simulink model "mcb_pmsm_foc_qep_dyno_f28069m_ADC"  (R2023b)
settings: Solver=FixedStepDiscrete  StartTime=0.0  StopTime=4  RelTol=1e-3  EnableMultiTasking=on
InitFcn:
  | mcb_pmsm_foc_qep_dyno_f28069m_data;
undefined symbols (not defined in the file): DiscIntNeverNeededParam, Down, GPTRIP1SEL, GPTRIP2SEL, inverter_motor1, inverter_motor2, PI_params_motor1, PI_params_motor2, pmsm_motor1, pmsm_motor2, PU_System_motor2, target, Ts, Ts_motor, Ts_speed, TZ1, TZ2, Up
libraries: c2802xlib x12, simulink x11, c280xlib x8, mcbcontrolslib x6, mcbpositiondecoderlib x6, c2806xlib x5, svdschedulerlib x3, mcbpmsmnonlinearlib x2, autolibpmsmexterior x2, mcbplantlib x2, demo_controls x1, slpidlib x1
(part 3 of 4)

== system mcb_pmsm_foc_qep_dyno_f28069m_ADC/Serial Receive/Code Generation ==
  SCI Receive : c280xlib/SCI Receive  sciModule=A  dataHead=''  headerCheckMaxCount=16  dataTail=''  dataType=uint16  dataLenOptions=Length via dialog  dataDim=2  maxDataLength=1  initValue=0  errOption=Output the last received value  errValue=0  sampleTime=-1  blockingMode=on  timeOut=0.019444  outputStatus=off
  Data : Outport
  wires:
  SCI Receive/1 -> Data/1

== system mcb_pmsm_foc_qep_dyno_f28069m_ADC/Serial Receive/Reference Signal ==
  In1 : Inport
  Data Store Write2 : DataStoreWrite  DataStoreName=Debug_signals  IndexOptions=Index vector (dialog)  Indices=1  OutputSizes=1
  Data_Conditioning : Subsystem
  If : If  IfExpression=u1 == 1  ElseIfExpressions=u1 == 2, u1 == 0  ShowElse=off
  If Action Subsystem : Subsystem  TreatAsAtomicUnit=on
  If Action Subsystem1 : Subsystem  TreatAsAtomicUnit=on
  If Action Subsystem2 : Subsystem  TreatAsAtomicUnit=on
  unParse : Subsystem
  Enable_PWM : Outport
  wires:
  If/3 -> If Action Subsystem2/Action
  unParse/3(Debug_sig) -> Data Store Write2/1
  Data_Conditioning/2(PU_data) -> If Action Subsystem2/1(In1), If Action Subsystem/1(In1), If Action Subsystem1/1(In1)
  If/2 -> If Action Subsystem1/Action
  If/1 -> If Action Subsystem/Action
  In1/1 -> Data_Conditioning/1(In1)
  unParse/2(Motor1/2) -> If/1
  Data_Conditioning/1(Logical signal) -> unParse/1(Data)
  unParse/1(Enable_PWM) -> Enable_PWM/1

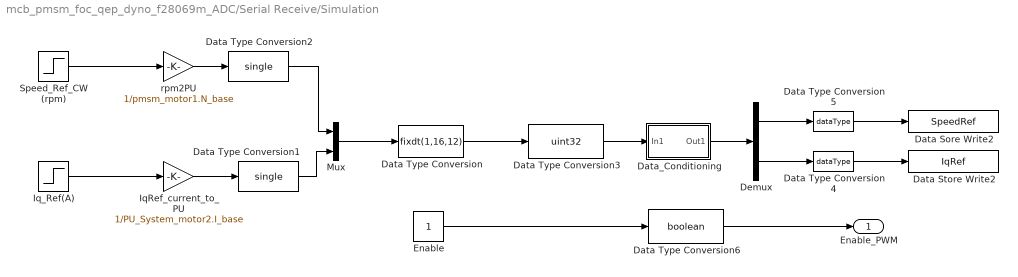
== system mcb_pmsm_foc_qep_dyno_f28069m_ADC/Serial Receive/Simulation ==
  Data Sore Write2 : DataStoreWrite  DataStoreName=SpeedRef  IndexOptions=Index vector (dialog)  Indices=1  OutputSizes=1
  Data Store Write2 : DataStoreWrite  DataStoreName=IqRef  IndexOptions=Index vector (dialog)  Indices=1  OutputSizes=1
  Data Type Conversion : DataTypeConversion  OutDataTypeStr=fixdt(1,16,12)  RndMeth=Simplest  SaturateOnIntegerOverflow=off
  Data Type Conversion1 : DataTypeConversion  OutDataTypeStr=single  RndMeth=Simplest  SaturateOnIntegerOverflow=off
  Data Type Conversion2 : DataTypeConversion  OutDataTypeStr=single  RndMeth=Simplest  SaturateOnIntegerOverflow=off
  Data Type Conversion3 : DataTypeConversion  OutDataTypeStr=uint32  ConvertRealWorld=Stored Integer (SI)  RndMeth=Simplest  SaturateOnIntegerOverflow=off
  Data Type Conversion4 : DataTypeConversion  OutDataTypeStr=dataType  RndMeth=Simplest  SaturateOnIntegerOverflow=off
  Data Type Conversion5 : DataTypeConversion  OutDataTypeStr=dataType  RndMeth=Simplest  SaturateOnIntegerOverflow=off
  Data Type Conversion6 : DataTypeConversion  OutDataTypeStr=boolean  SaturateOnIntegerOverflow=off  RndMeth=Floor
  Data_Conditioning : Subsystem
  Demux : Demux  Outputs=2
  Enable : Constant  OutDataTypeStr=single
  IqRef_current_to_PU : Gain  Gain=1/PU_System_motor2.I_base  RndMeth=Simplest  OutDataTypeStr=Inherit: Same as input
  Iq_Ref(A) : Step  Time=3  Before=1  After=0.8*pmsm_motor2.I_rated  OutDataTypeStr=single
  Mux : Mux  Inputs=2
  Speed_Ref_CW (rpm) : Step  Before=0.2*pmsm_motor1.N_base  After=0.5*pmsm_motor1.N_base  OutDataTypeStr=single
  rpm2PU : Gain  Gain=1/pmsm_motor1.N_base  RndMeth=Simplest  OutDataTypeStr=Inherit: Same as input
  Enable_PWM : Outport
  wires:
  Data Type Conversion3/1 -> Data_Conditioning/1(In1)
  rpm2PU/1 -> Data Type Conversion2/1
  Data Type Conversion1/1 -> Mux/2
  Data Type Conversion2/1 -> Mux/1
  Data Type Conversion/1 -> Data Type Conversion3/1
  Mux/1 -> Data Type Conversion/1
  Speed_Ref_CW (rpm)/1 -> rpm2PU/1
  IqRef_current_to_PU/1 -> Data Type Conversion1/1
  Iq_Ref(A)/1 -> IqRef_current_to_PU/1
  Data_Conditioning/1(Out1) -> Demux/1
  Demux/1 -> Data Type Conversion5/1
  Data Type Conversion4/1 -> Data Store Write2/1
  Demux/2 -> Data Type Conversion4/1
  Data Type Conversion5/1 -> Data Sore Write2/1
  Data Type Conversion6/1 -> Enable_PWM/1
  Enable/1 -> Data Type Conversion6/1

== system mcb_pmsm_foc_qep_dyno_f28069m_ADC/Simulation/Simulation1 ==
  Trigger : TriggerPort  VariantControl=Variant  PortDimensions=1
  ADCINT1 : simulink/Ports & Subsystems/Function-Call Generator  sample_time=-1  numberOfIterations=1  DisallowWideOutput=off
  Interrupt : Outport
  wires:
  ADCINT1/1 -> Interrupt/1

== system mcb_pmsm_foc_qep_dyno_f28069m_ADC/Simulation/Simulation2 ==
  Trigger : TriggerPort  VariantControl=Variant  PortDimensions=1
  ADCINT1 : simulink/Ports & Subsystems/Function-Call Generator  sample_time=-1  numberOfIterations=1  DisallowWideOutput=off
  Interrupt : Outport
  wires:
  ADCINT1/1 -> Interrupt/1

== system mcb_pmsm_foc_qep_dyno_f28069m_ADC/Speed Control for motor1/PI_Controller_Speed ==
  N_ref : Inport
  N_fb : Inport  Port=2
  AND : Logic  IconShape=distinctive  AllPortsSameDT=off  OutDataTypeStr=boolean
  Data Store Read1 : DataStoreRead  DataStoreName=Enable  IndexOptions=Index vector (dialog)  Indices=1  OutputSizes=1
  Data Store Read2 : DataStoreRead  DataStoreName=EnClosedLoop  IndexOptions=Index vector (dialog)  Indices=1  OutputSizes=1
  Discrete PI Controller with anti-windup & reset : slpidlib/PID Controller  Controller=PI  Form=Parallel  TimeDomain=Discrete-time  UseExternalTs=off  SampleTime=-1  IntegratorMethod=Forward Euler  FilterMethod=Forward Euler  ControllerParametersSource=external  P=1  I=1  UseKiTs=on  D=0  N=100  UseFilter=on  TunerSelectOption=Transfer Function Based (PID Tuner App)  InitialConditionSource=external  InitialConditionForIntegrator=0  InitialConditionForFilter=0  DifferentiatorICPrevScaledInput=0  ExternalReset=level  TrackingMode=off  Kt=1  LimitOutput=on  SatLimitsSource=internal  UpperSaturationLimit=1  LowerSaturationLimit=-1  LinearizeAsGain=on  AntiWindupMode=clamping  Kb=1  LimitIntegrator=off  UpperIntegratorSaturationLimit=inf  LowerIntegratorSaturationLimit=-inf  RndMeth=Simplest  POutMin=[]  POutMax=[]  IOutMin=[]  IOutMax=[]  DOutMin=[]  DOutMax=[]  NOutMin=[]  NOutMax=[]  SumOutMin=[]  SumOutMax=[]  SaturationOutDataTypeStr=Inherit: Inherit via back propagation  SaturationOutMin=[]  SaturationOutMax=[]  PParamMin=[]  PParamMax=[]  IParamMin=[]  IParamMax=[]  DParamMin=[]  DParamMax=[]  NParamMin=[]  NParamMax=[]  KbParamMin=[]  KbParamMax=[]  KtParamMin=[]  KtParamMax=[]  KbOutMin=[]  KbOutMax=[]  KtOutMin=[]  KtOutMax=[]  IntegratorOutMin=[]  IntegratorOutMax=[]  FilterOutMin=[]  FilterOutMax=[]  SumI1OutMin=[]  SumI1OutMax=[]  SumI2OutMin=[]  SumI2OutMax=[]  SumI3OutMin=[]  SumI3OutMax=[]  SumI4OutMin=[]  SumI4OutMax=[]  SumDOutMin=[]  SumDOutMax=[]  DifferentiatorOutMin=[]  DifferentiatorOutMax=[]  FilterDiffOutCoefMin=[]  FilterDiffOutCoefMax=[]  ReciprocalOutMin=[]  ReciprocalOutMax=[]  SumDenOutMin=[]  SumDenOutMax=[]  SumNumOutMin=[]  SumNumOutMax=[]  DivideOutMin=[]  DivideOutMax=[]  UdiffTsProdOutMin=[]  UdiffTsProdOutMax=[]  NTsProdOutMin=[]  NTsProdOutMax=[]  UintegralTsProdOutMin=[]  UintegralTsProdOutMax=[]  UngainTsProdOutMin=[]  UngainTsProdOutMax=[]  ClampingZeroOutDataTypeStr=Inherit: Inherit via back propagation  ClampingZeroOutMin=[]  ClampingZeroOutMax=[]  FilterDenConstantOutDataTypeStr=Inherit: Inherit via back propagation  FilterDenConstantOutMin=[]  FilterDenConstantOutMax=[]  PCopyOutDataTypeStr=Inherit: Inherit via back propagation  PCopyOutMin=[]  PCopyOutMax=[]  NCopyOutDataTypeStr=Inherit: Inherit via back propagation  NCopyOutMin=[]  NCopyOutMax=[]  IntegratorContinuousStateAttributes=''  IntegratorStateMustResolveToSignalObject=off  IntegratorRTWStateStorageClass=Auto  FilterContinuousStateAttributes=''  FilterStateMustResolveToSignalObject=off  FilterRTWStateStorageClass=Auto  ParallelPVariant=ExternalParameters  IdealPVariant=Disabled  IVariant=ExternalParameters  DVariant=Disabled  IntegratorVariant=Discrete  SatVariant=Enabled  AWVariant=DiscClampingParallel  PCopyVariant=Disabled  TRVariant=Disabled  FdbkBlocksVariant=Forward  IdealPFdbkVariant=Disabled  SatFdbkVariant=Disabled  DerivativeFilterVariant=Disabled  NVariant=Disabled  NCopyVariant=Disabled_SignalSpec  FilterICVariant=Disabled  IntegratorICVariant=ExternalICs  ExternalResetVariant=ExternalReset  TRSumVariant=Passthrough  SumFdbkVariant=Disabled  SumVariant=Sum_PI  TsampFilterVariant=InternalTs  TsampNgainVariant=Passthrough  TsampIntegralVariant=Disabled_SignalSpec  ExternalSaturationOutDataTypeStr=Inherit: Same as second input
  Ki1 : Constant  Value=PI_params_motor1.Ki_speed*Ts_speed  OutDataTypeStr=dataType  SampleTime=-1
  Ki2 : Constant  Value=0  OutDataTypeStr=dataType  SampleTime=-1
  Kp1 : Constant  Value=PI_params_motor1.Kp_speed  OutDataTypeStr=dataType  SampleTime=-1
  Logical Operator : Logic  Operator=NOT  IconShape=distinctive  AllPortsSameDT=off  OutDataTypeStr=boolean
  Sum : Sum  Inputs=|+-  OutDataTypeStr=Inherit: Same as first input
  Iq_ref : Outport  VectorParamsAs1DForOutWhenUnconnected=off
  wires:
  Discrete PI Controller with anti-windup & reset/1 -> Iq_ref/1
  Ki1/1 -> Discrete PI Controller with anti-windup & reset/3
  Kp1/1 -> Discrete PI Controller with anti-windup & reset/2
  N_fb/1 -> Sum/2
  N_ref/1 -> Sum/1
  Sum/1 -> Discrete PI Controller with anti-windup & reset/1
  Logical Operator/1 -> Discrete PI Controller with anti-windup & reset/4
  Ki2/1 -> Discrete PI Controller with anti-windup & reset/5
  AND/1 -> Logical Operator/1
  Data Store Read1/1 -> AND/1
  Data Store Read2/1 -> AND/2

== system mcb_pmsm_foc_qep_dyno_f28069m_ADC/Speed Control for motor1/Speed_Ref_Selector ==
  Speed_Ref_In : Inport
  Speed_Ref_Open : Inport  Port=2
  Data Store Read : DataStoreRead  DataStoreName=EnClosedLoop  IndexOptions=Index vector (dialog)  Indices=1  OutputSizes=1
  IIR Filter : mcbcontrolslib/IIR Filter  VariantControl=Low Pass Filter  VariantSelect=Low-pass  Filter_constant=0.01  advancedSettings=off  Ts=50e-6  cutOff_freq=32.1525
  Switch : Switch  Criteria=u2 > Threshold  Threshold=0.5  SaturateOnIntegerOverflow=off  InputSameDT=off
  Speed_Ref_PU : Outport
  wires:
  IIR Filter/1 -> Speed_Ref_PU/1
  Switch/1 -> IIR Filter/1
  Data Store Read/1 -> Switch/2
  Speed_Ref_Open/1 -> Switch/3
  Speed_Ref_In/1 -> Switch/1

== system mcb_pmsm_foc_qep_dyno_f28069m_ADC/FOC Algorithm Motor1/Control_System/Closed loop Control ==
  Iab_meas_PU : Inport
  Pos_PU : Inport  Port=2
  Idq_ref_PU : Inport  Port=3
  EnablePWM : Inport  Port=4
  Enable : EnablePort
  Current Control : Subsystem  ReferencedSubsystem=current_control  Kpd=PI_params_motor1.Kp_i  Kid=PI_params_motor1.Ki_i*Ts  Kpq=PI_params_motor1.Kp_i  Kiq=PI_params_motor1.Ki_i*Ts
  Terminator : Terminator
  Vabc in PU : Outport
  Idq_debug : Outport  Port=2
  wires:
  Current Control/1 -> Vabc in PU/1
  Idq_ref_PU/1 -> Current Control/3
  EnablePWM/1 -> Current Control/4
  Current Control/2 -> Idq_debug/1
  Pos_PU/1 -> Current Control/2
  Iab_meas_PU/1 -> Current Control/1
  Current Control/3 -> Terminator/1

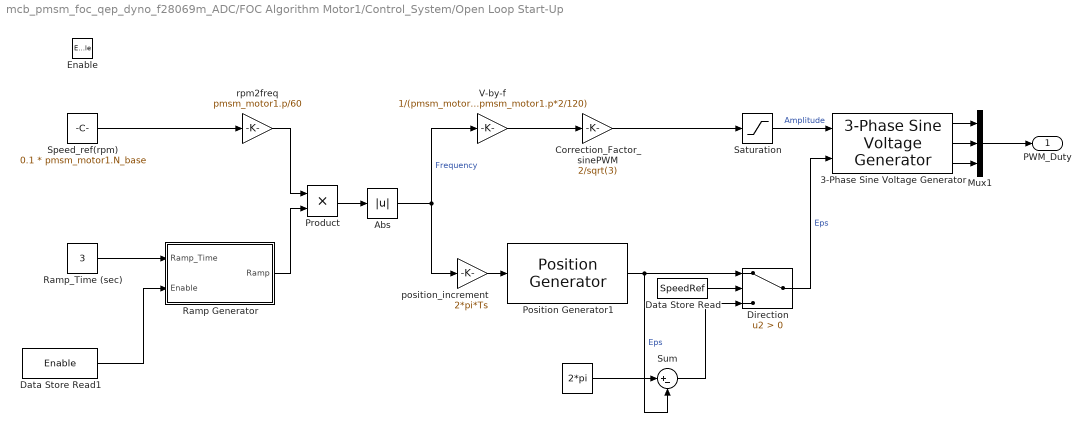
== system mcb_pmsm_foc_qep_dyno_f28069m_ADC/FOC Algorithm Motor1/Control_System/Open Loop Start-Up ==
  Enable : EnablePort
  " " : Constant  Value=2*pi  OutDataTypeStr=dataType  SampleTime=-1
  3-Phase Sine Voltage Generator : mcbcontrolslib/3-Phase Sine Voltage Generator  AngleInput=Radians  N_points=1024
  Abs : Abs  SaturateOnIntegerOverflow=off
  Correction_Factor_sinePWM : Gain  Gain=2/sqrt(3)  RndMeth=Simplest  OutDataTypeStr=Inherit: Same as input
  Data Store Read : DataStoreRead  DataStoreName=SpeedRef  IndexOptions=Index vector (dialog)  Indices=1  OutputSizes=1
  Data Store Read1 : DataStoreRead  DataStoreName=Enable  IndexOptions=Index vector (dialog)  Indices=1  OutputSizes=1
  Direction : Switch  Criteria=u2 > Threshold  OutDataTypeStr=dataType  RndMeth=Simplest  SaturateOnIntegerOverflow=off  InputSameDT=off
  Mux1 : Mux  Inputs=3
  Position Generator1 : mcbcontrolslib/Position Generator  AngleOutput=Radians  ExternalReset=none  Offset=0
  Product : Product  RndMeth=Simplest  OutDataTypeStr=Inherit: Same as first input
  Ramp Generator : Subsystem
  Ramp_Time (sec) : Constant  Value=3  OutDataTypeStr=dataType  SampleTime=-1
  Saturation : Saturate  UpperLimit=0.95  LowerLimit=0.15  RndMeth=Simplest
  Speed_ref(rpm) : Constant  Value=0.1 * pmsm_motor1.N_base  OutDataTypeStr=dataType  SampleTime=-1
  Sum : Sum  Inputs=|+-  RndMeth=Simplest  OutDataTypeStr=Inherit: Same as first input
  V-by-f : Gain  Gain=1/(pmsm_motor1.N_base*pmsm_motor1.p*2/120)  RndMeth=Simplest  OutDataTypeStr=Inherit: Same as input
  position_increment : Gain  Gain=2*pi*Ts  RndMeth=Simplest  OutDataTypeStr=Inherit: Same as input
  rpm2freq : Gain  Gain=pmsm_motor1.p/60  RndMeth=Simplest  OutDataTypeStr=Inherit: Same as input
  PWM_Duty : Outport  VectorParamsAs1DForOutWhenUnconnected=off
  wires:
  3-Phase Sine Voltage Generator/1 -> Mux1/1
  3-Phase Sine Voltage Generator/3 -> Mux1/3
  Direction/1 -> 3-Phase Sine Voltage Generator/2  "Eps"
  Speed_ref(rpm)/1 -> rpm2freq/1
  Saturation/1 -> 3-Phase Sine Voltage Generator/1  "Amplitude"
  Mux1/1 -> PWM_Duty/1
  Ramp Generator/1(Ramp) -> Product/2
  Ramp_Time (sec)/1 -> Ramp Generator/1(Ramp_Time)
  Position Generator1/1 -> Sum/2, Direction/1  "Eps"
  " "/1 -> Sum/1
  Sum/1 -> Direction/3
  Abs/1 -> position_increment/1, V-by-f/1  "Frequency"
  position_increment/1 -> Position Generator1/1
  V-by-f/1 -> Correction_Factor_sinePWM/1
  Product/1 -> Abs/1
  rpm2freq/1 -> Product/1
  Correction_Factor_sinePWM/1 -> Saturation/1
  3-Phase Sine Voltage Generator/2 -> Mux1/2
  Data Store Read1/1 -> Ramp Generator/2(Enable)
  Data Store Read/1 -> Direction/2

== system mcb_pmsm_foc_qep_dyno_f28069m_ADC/FOC Algorithm Motor1/HW_Inputs/Sensor Driver Blocks (codegen) ==
  Sim : Inport
  IA/IB Measurement : c2802xlib/ADC  blkParamProc=C2000  ADCModule=1  samplingMode=Simultaneous sample mode  ADCResolution=12-bit (Single-ended input)  useSOC1=SOC0  useSOC2=SOC0_SOC1  SOCAcquisitionWindow=7  SOCTriggerSource=ePWM1_ADCSOCA  SOCInterruptTrigger=No ADCINT  Ts=-1  dType=uint16  postInterrupt=on  interruptSel=ADCINT1  ADCINTContinuous=on  endma=off  chdma=1  conv1=ADCINB1  conv2=ADCINA0 and ADCINB0  conv1_Type4=ADCIN0  conv2_Type4=ADCIN0 and ADCIN1
  IA/IB Measurement3 : c2802xlib/ADC  blkParamProc=C2000  ADCModule=1  samplingMode=Simultaneous sample mode  ADCResolution=12-bit (Single-ended input)  useSOC1=SOC0  useSOC2=SOC12_SOC13  SOCAcquisitionWindow=8  SOCTriggerSource=ePWM1_ADCSOCA  SOCInterruptTrigger=No ADCINT  Ts=-1  dType=uint16  postInterrupt=on  interruptSel=ADCINT5  ADCINTContinuous=on  endma=off  chdma=1  conv1=ADCINB1  conv2=ADCINA2 and ADCINB2  conv1_Type4=ADCIN0  conv2_Type4=ADCIN0 and ADCIN1
  IC/VA Measurement : c2802xlib/ADC  blkParamProc=C2000  ADCModule=1  samplingMode=Simultaneous sample mode  ADCResolution=12-bit (Single-ended input)  useSOC1=SOC0  useSOC2=SOC14_SOC15  SOCAcquisitionWindow=7  SOCTriggerSource=ePWM1_ADCSOCA  SOCInterruptTrigger=No ADCINT  Ts=-1  dType=uint16  postInterrupt=on  interruptSel=ADCINT9  ADCINTContinuous=on  endma=off  chdma=1  conv1=ADCINB1  conv2=ADCINA1 and ADCINB1  conv1_Type4=ADCIN0  conv2_Type4=ADCIN0 and ADCIN1
  Mux : Mux  Inputs=3
  Terminator : Terminator
  eQEP : c280xlib/eQEP  useModule=eQEP1  pcInputmode=Quadrature-count  externalClockrate=2x resolution: Count the rising/falling edge  swapPolarityselection=Clockwise  qdfOutputport=off  qapPolarityselection=on  qbpPolarityselection=on  qipPolarityselection=on  qspPolarityselection=off  igatePolarityselection=off  sampleTime=-1  pcOutputport=on  pcMaximumvalue=2^16-1  indexInitializationcheck=off  indexInitializationevent=Falling edge  strobeInitializationcheck=off  strobeInitializationevent=Rising edge  softwareInitializationcheck=off  softwareInitializationsource=Set to init value at start up  softwareInitializationmode=on  pcInitialvalue=0  pcResetmode=Reset on the first index event  ieloutputport=on  indexEventlatch=Falling edge  seloutputport=off  strobeEventlatch=Rising edge  pcefOutputport=off  enableEqepcapture=off  qctmrOutputport=off  qcprdOutputport=off  captureTimerprescaler=128  upEventprescaler=128  overflowErrorflag=off  directionErrorflag=off  captureTimerposition=On position counter read  unitTimerperiod=100000000  captureTimerlatch=off  capturePeriodlatch=off  positionCounterlatch=off  soenPolarityselection=off  spselPolarityselection=Index pin is used for sync output  compareValuesource=Specify via dialog  shadowMode=Load on QPOSCNT=0  compareValue=4294967295  syncOutputwidth=1  polaritySyncoutput=Active high  watchdogEnable=off  watchdogTimer=65535  outport1Datatype=auto  outport2Datatype=auto  outport3Datatype=auto  outport4Datatype=auto  outport5Datatype=auto  outport6Datatype=auto  outport7Datatype=auto  outport8Datatype=auto  outport9Datatype=auto  outport10Datatype=auto  outport11Datatype=auto  outport12Datatype=auto  eqepinterrupt_pce=off  eqepinterrupt_qpe=off  eqepinterrupt_qdc=off  eqepinterrupt_wto=off  eqepinterrupt_pcu=off  eqepinterrupt_pco=off  eqepinterrupt_pcr=off  eqepinterrupt_pcm=off  eqepinterrupt_sel=off  eqepinterrupt_iel=off  eqepinterrupt_uto=off  pheOutputport=off  watchdogOutputport=off  outport13Datatype=auto  outport14Datatype=auto
  out : Outport
  I_A1 and I_B1 : Outport  Port=2
  I_C1 and V_A1 : Outport  Port=3
  V_B1 and V_C1 : Outport  Port=4
  wires:
  Sim/1 -> Terminator/1
  Mux/1 -> out/1
  eQEP/1 -> Mux/2
  eQEP/2 -> Mux/3
  IA/IB Measurement/1 -> I_A1 and I_B1/1, Mux/1
  IC/VA Measurement/1 -> I_C1 and V_A1/1
  IA/IB Measurement3/1 -> V_B1 and V_C1/1

== system mcb_pmsm_foc_qep_dyno_f28069m_ADC/FOC Algorithm Motor1/HW_Inputs/Sensor Driver Blocks (sim) ==
  Sim : Inport
  out : Outport
  wires:
  Sim/1 -> out/1

== system mcb_pmsm_foc_qep_dyno_f28069m_ADC/FOC Algorithm Motor1/Input Scaling/ Calculate Speed ==
  QEP_Position_Count : Inport
  QEP_Index_Latch : Inport  Port=2
  Offset : Inport  Port=3
  Delay : Delay  DelayLength=1
  IIR Filter : mcbcontrolslib/IIR Filter  VariantControl=Low Pass Filter  VariantSelect=Low-pass  Filter_constant=0.01  advancedSettings=off  Ts=50e-6  cutOff_freq=32.1525
  IndexFinder : Subsystem
  Mechanical to Electrical Position : mcbpositiondecoderlib/Mechanical to Electrical Position  PolePairsInputType=Specify via dialog  NrPP=pmsm_motor1.p  selectedRange=Per unit  MechOfstInputType=Input port  mechOffsetIn=0  maxAngleIn=1  InputDataType=dataType  VariantSelect=floating-point
  NOT : Logic  Operator=NOT  AllPortsSameDT=off  OutDataTypeStr=boolean
  Quadrature Decoder : mcbpositiondecoderlib/Quadrature Decoder  EncoderSlitsPerRevolution=pmsm_motor1.QEPSlits  EncoderCountsPerSlit=4  CounterSize=16 bits  ExternalIndexCount=on  PositionUnit=Per unit  PositionDataType=dataType  ParameterInputType=off  CountsPerRevInverseDataType=single
  Speed Measurement : mcbpositiondecoderlib/Speed Measurement  PositionUnit=Per unit  PositionScalingDatatype=uint32  SpeedCalculationMode=Time interval for speed calculation  SampleTimeAsync=Ts  MaximumApplicationSpeed=6000  SpeedResolution=5e-6  DelayLength=20  MaximumMeasurableSpeed=14999  MeasurableSpeedResolution=6.9849e-06  SpeedUnit=Per unit based on dialog  PerUnitSpeed=pmsm_motor1.N_base  SpeedDataType=dataType
  Theta_e : Outport  VectorParamsAs1DForOutWhenUnconnected=off
  speed : Outport  Port=2  VectorParamsAs1DForOutWhenUnconnected=off
  IndexFound : Outport  Port=3  InitialOutput=0  VectorParamsAs1DForOutWhenUnconnected=off
  wires:
  Mechanical to Electrical Position/1 -> Theta_e/1
  Speed Measurement/1 -> IIR Filter/1
  Quadrature Decoder/1 -> Speed Measurement/1, Mechanical to Electrical Position/1
  QEP_Position_Count/1 -> Quadrature Decoder/1
  Offset/1 -> Mechanical to Electrical Position/2
  IIR Filter/1 -> speed/1
  NOT/1 -> IndexFinder/Enable
  IndexFinder/1(Out1) -> Delay/1, IndexFound/1
  QEP_Index_Latch/1 -> IndexFinder/1(In1), Quadrature Decoder/2
  Delay/1 -> NOT/1

== system mcb_pmsm_foc_qep_dyno_f28069m_ADC/FOC Algorithm Motor1/Input Scaling/Calculate Phase Currents ==
  Ia_ADC : Inport
  Ib_ADC : Inport  Port=2
  Add : Sum  Inputs=-+
  Data Store Read : DataStoreRead  DataStoreName=IaOffset_motor1  IndexOptions=Index vector (dialog)  Indices=1  OutputSizes=1
  Data Store Read1 : DataStoreRead  DataStoreName=IbOffset_motor1  IndexOptions=Index vector (dialog)  Indices=1  OutputSizes=1
  Data Type Conversion : DataTypeConversion  OutDataTypeStr=int32  ConvertRealWorld=Stored Integer (SI)  SaturateOnIntegerOverflow=off  RndMeth=Floor
  Data Type Conversion1 : DataTypeConversion  OutDataTypeStr=dataType  SaturateOnIntegerOverflow=off  RndMeth=Floor
  Data Type Conversion3 : DataTypeConversion  OutDataTypeStr=fixdt(1,32,17)  ConvertRealWorld=Stored Integer (SI)  RndMeth=Simplest  SaturateOnIntegerOverflow=off
  Inverting / Non-inverting Current measurement amplifier : Gain  Gain=inverter_motor1.invertingAmp  RndMeth=Simplest  OutDataTypeStr=Inherit: Same as input
  Mux : Mux  Inputs=2
  Mux1 : Mux  Inputs=2
  Q17 per unit conversion : ArithShift  BitShiftNumber=-6
  Iab_meas_PU : Outport  VectorParamsAs1DForOutWhenUnconnected=off
  wires:
  Mux1/1 -> Add/1
  Data Type Conversion/1 -> Add/2
  Q17 per unit conversion/1 -> Data Type Conversion3/1
  Ia_ADC/1 -> Mux/1
  Add/1 -> Q17 per unit conversion/1
  Ib_ADC/1 -> Mux/2
  Mux/1 -> Data Type Conversion/1
  Data Type Conversion1/1 -> Inverting / Non-inverting Current measurement amplifier/1
  Data Type Conversion3/1 -> Data Type Conversion1/1
  Data Store Read/1 -> Mux1/1
  Data Store Read1/1 -> Mux1/2
  Inverting / Non-inverting Current measurement amplifier/1 -> Iab_meas_PU/1

== system mcb_pmsm_foc_qep_dyno_f28069m_ADC/FOC Algorithm Motor1/SCI (Code Generation)/Data_Logging ==
  note: Fast Serial Data Monitoring (32-bit)
  Data_Log1 : Inport
  Data_Log2 : Inport  Port=2
  Counter Limited : simulink/Sources/Counter Limited  uplimit=599  tsamp=-1
  Data : Subsystem  TreatAsAtomicUnit=on
  Data_Conditioning : Subsystem
  End : Subsystem  TreatAsAtomicUnit=on
  If : If  IfExpression=u1 == 0  ElseIfExpressions=u1 == 599
  Merge : Merge  Inputs=3
  Merge1 : Merge  Inputs=3
  Mux : Mux  Inputs=2
  Mux3 : Mux  Inputs=2
  Start : Subsystem  TreatAsAtomicUnit=on
  Width : Width  OutDataTypeMode=All ports same datatype  DataType=uint16
  SCI_Tx : Outport
  wires:
  If/3 -> Data/Action
  Data/1(Data_out) -> Merge/3
  Width/1 -> Data/2(Data_width), Start/2(Data_width), End/2(Data_width)
  Merge/1 -> Mux/1  "SCI_Tx_Data"
  Counter Limited/1 -> If/1
  Start/2(Iteration) -> Merge1/1
  Start/1(Data_out) -> Merge/1
  If/2 -> End/Action
  Merge1/1 -> Mux/2  "SCI_Tx_Iteration"
  If/1 -> Start/Action
  End/1(Data_out) -> Merge/2
  End/2(Iteration) -> Merge1/2
  Data/2(Iteration) -> Merge1/3
  Data_Log1/1 -> Mux3/1
  Data_Conditioning/1(Out1) -> Width/1, Start/1(Data), End/1(Data), Data/1(Data)
  Mux/1 -> SCI_Tx/1
  Mux3/1 -> Data_Conditioning/1(In1)
  Data_Log2/1 -> Mux3/2

== system mcb_pmsm_foc_qep_dyno_f28069m_ADC/FOC Algorithm Motor1/SCI (Code Generation)/While Iterator Subsystem ==
  Data : Inport
  Iteration : Inport  Port=2
  Add : Sum  Inputs=+-  OutDataTypeStr=Inherit: Same as first input
  Index Vector : MultiPortSwitch  Inputs=1  SaturateOnIntegerOverflow=off  InputSameDT=off
  SCI Transmit : c280xlib/SCI Transmit  sciModule=A  dataHead=''  dataTail=''  frameSize=1  blockingMode=on  outputStatus=off
  While Iterator : WhileIterator  MaxIters=-1  WhileBlockType=do-while  ShowIterationPort=on  OutputDataType=int16
  wires:
  While Iterator/1 -> Add/2, Index Vector/1
  Data/1 -> Index Vector/2
  Index Vector/1 -> SCI Transmit/1
  Add/1 -> While Iterator/1
  Iteration/1 -> Add/1

== system mcb_pmsm_foc_qep_dyno_f28069m_ADC/FOC Algorithm Motor2/Control_System/Closed loop ==
  Iab_meas_PU : Inport
  Pos_PU : Inport  Port=2
  Idq_ref_PU : Inport  Port=3
  EnablePWM : Inport  Port=4
  Enable : EnablePort
  Current Control : Subsystem  ReferencedSubsystem=current_control  Kpd=PI_params_motor2.Kp_i  Kid=PI_params_motor2.Ki_i*Ts  Kpq=PI_params_motor2.Kp_i  Kiq=PI_params_motor2.Ki_i*Ts
  Terminator : Terminator
  Vabc in PU : Outport
  Idq_debug : Outport  Port=2
  wires:
  Iab_meas_PU/1 -> Current Control/1
  Idq_ref_PU/1 -> Current Control/3
  Pos_PU/1 -> Current Control/2
  Current Control/1 -> Vabc in PU/1
  Current Control/2 -> Idq_debug/1
  EnablePWM/1 -> Current Control/4
  Current Control/3 -> Terminator/1

== system mcb_pmsm_foc_qep_dyno_f28069m_ADC/FOC Algorithm Motor2/Enable Motor2 after a delay/Delay to start motor1 (codegen) ==
  note: Add 2 seconds delay from Enable and Closed-loop enable.
      | This ensures motor with speed control starts and settles before
      | motor with torque control starts.
  AND : Logic  IconShape=distinctive  AllPortsSameDT=off  OutDataTypeStr=boolean
  Data Store Read1 : DataStoreRead  DataStoreName=Enable  IndexOptions=Index vector (dialog)  Indices=1  OutputSizes=1
  Data Store Read2 : DataStoreRead  DataStoreName=EnClosedLoop  IndexOptions=Index vector (dialog)  Indices=1  OutputSizes=1
  Disable EnMtr2TrqCtrl : Subsystem  TreatAsAtomicUnit=on
  Enable EnMtr2TrqCtrl after 2 sec delay : Subsystem  TreatAsAtomicUnit=on
  NOT : Logic  Operator=NOT  IconShape=distinctive  AllPortsSameDT=off  OutDataTypeStr=boolean
  wires:
  AND/1 -> NOT/1, Enable EnMtr2TrqCtrl after 2 sec delay/Enable
  NOT/1 -> Disable EnMtr2TrqCtrl/Enable
  Data Store Read2/1 -> AND/1
  Data Store Read1/1 -> AND/2

== system mcb_pmsm_foc_qep_dyno_f28069m_ADC/FOC Algorithm Motor2/Enable Motor2 after a delay/Delay to start motor2 (sim) ==
  note: In simulation, delay 0.5 second after Enable and EnClosedLoop (Index found).
  AND1 : Logic  IconShape=distinctive  AllPortsSameDT=off  OutDataTypeStr=boolean
  Data Store Read3 : DataStoreRead  DataStoreName=Enable  IndexOptions=Index vector (dialog)  Indices=1  OutputSizes=1
  Data Store Read4 : DataStoreRead  DataStoreName=EnClosedLoop  IndexOptions=Index vector (dialog)  Indices=1  OutputSizes=1
  Delay 0.5 sec : Subsystem  TreatAsAtomicUnit=on
  Enabled Subsystem : Subsystem  TreatAsAtomicUnit=on
  Enabled Subsystem2 : Subsystem  TreatAsAtomicUnit=on
  NOT : Logic  Operator=NOT  IconShape=distinctive  AllPortsSameDT=off  OutDataTypeStr=boolean
  wires:
  Data Store Read4/1 -> AND1/1
  NOT/1 -> Enabled Subsystem2/Enable
  Delay 0.5 sec/1(Out1) -> Enabled Subsystem/Enable
  AND1/1 -> NOT/1, Delay 0.5 sec/Enable
  Data Store Read3/1 -> AND1/2

== system mcb_pmsm_foc_qep_dyno_f28069m_ADC/FOC Algorithm Motor2/HW_Inputs1/Sensor Driver Blocks (codegen) ==
  Sim : Inport
  IA/IB Measurement : c2802xlib/ADC  blkParamProc=C2000  ADCModule=1  samplingMode=Simultaneous sample mode  ADCResolution=12-bit (Single-ended input)  useSOC1=SOC0  useSOC2=SOC2_SOC3  SOCAcquisitionWindow=7  SOCTriggerSource=ePWM4_ADCSOCA  SOCInterruptTrigger=No ADCINT  Ts=-1  dType=uint16  postInterrupt=on  interruptSel=ADCINT2  ADCINTContinuous=on  endma=off  chdma=1  conv1=ADCINB1  conv2=ADCINA3 and ADCINB3  conv1_Type4=ADCIN0  conv2_Type4=ADCIN0 and ADCIN1
  Mux : Mux  Inputs=3
  Terminator : Terminator
  eQEP : c280xlib/eQEP  useModule=eQEP2  pcInputmode=Quadrature-count  externalClockrate=2x resolution: Count the rising/falling edge  swapPolarityselection=Clockwise  qdfOutputport=off  qapPolarityselection=on  qbpPolarityselection=on  qipPolarityselection=on  qspPolarityselection=off  igatePolarityselection=off  sampleTime=-1  pcOutputport=on  pcMaximumvalue=2^16-1  indexInitializationcheck=off  indexInitializationevent=Falling edge  strobeInitializationcheck=off  strobeInitializationevent=Rising edge  softwareInitializationcheck=off  softwareInitializationsource=Set to init value at start up  softwareInitializationmode=on  pcInitialvalue=0  pcResetmode=Reset on the first index event  ieloutputport=on  indexEventlatch=Falling edge  seloutputport=off  strobeEventlatch=Rising edge  pcefOutputport=off  enableEqepcapture=off  qctmrOutputport=off  qcprdOutputport=off  captureTimerprescaler=128  upEventprescaler=128  overflowErrorflag=off  directionErrorflag=off  captureTimerposition=On position counter read  unitTimerperiod=100000000  captureTimerlatch=off  capturePeriodlatch=off  positionCounterlatch=off  soenPolarityselection=off  spselPolarityselection=Index pin is used for sync output  compareValuesource=Specify via dialog  shadowMode=Load on QPOSCNT=0  compareValue=4294967295  syncOutputwidth=1  polaritySyncoutput=Active high  watchdogEnable=off  watchdogTimer=65535  outport1Datatype=auto  outport2Datatype=auto  outport3Datatype=auto  outport4Datatype=auto  outport5Datatype=auto  outport6Datatype=auto  outport7Datatype=auto  outport8Datatype=auto  outport9Datatype=auto  outport10Datatype=auto  outport11Datatype=auto  outport12Datatype=auto  eqepinterrupt_pce=off  eqepinterrupt_qpe=off  eqepinterrupt_qdc=off  eqepinterrupt_wto=off  eqepinterrupt_pcu=off  eqepinterrupt_pco=off  eqepinterrupt_pcr=off  eqepinterrupt_pcm=off  eqepinterrupt_sel=off  eqepinterrupt_iel=off  eqepinterrupt_uto=off  pheOutputport=off  watchdogOutputport=off  outport13Datatype=auto  outport14Datatype=auto
  out : Outport
  wires:
  Sim/1 -> Terminator/1
  IA/IB Measurement/1 -> Mux/1
  Mux/1 -> out/1
  eQEP/1 -> Mux/2
  eQEP/2 -> Mux/3

== system mcb_pmsm_foc_qep_dyno_f28069m_ADC/FOC Algorithm Motor2/HW_Inputs1/Sensor Driver Blocks (sim) ==
  Sim : Inport
  out : Outport
  wires:
  Sim/1 -> out/1

== system mcb_pmsm_foc_qep_dyno_f28069m_ADC/FOC Algorithm Motor2/Input Scaling/ Calculate Speed ==
  QEP_Position_Count : Inport
  QEP_Index_Latch : Inport  Port=2
  Offset : Inport  Port=3
  Delay : Delay  DelayLength=1
  IIR Filter : mcbcontrolslib/IIR Filter  VariantControl=Low Pass Filter  VariantSelect=Low-pass  Filter_constant=0.01  advancedSettings=off  Ts=50e-6  cutOff_freq=32.1525
  IndexFinder : Subsystem
  Mechanical to Electrical Position : mcbpositiondecoderlib/Mechanical to Electrical Position  PolePairsInputType=Specify via dialog  NrPP=pmsm_motor2.p  selectedRange=Per unit  MechOfstInputType=Input port  mechOffsetIn=0  maxAngleIn=1  InputDataType=dataType  VariantSelect=floating-point
  NOT : Logic  Operator=NOT  AllPortsSameDT=off  OutDataTypeStr=boolean
  Quadrature Decoder : mcbpositiondecoderlib/Quadrature Decoder  EncoderSlitsPerRevolution=pmsm_motor2.QEPSlits  EncoderCountsPerSlit=4  CounterSize=16 bits  ExternalIndexCount=on  PositionUnit=Per unit  PositionDataType=dataType  ParameterInputType=off  CountsPerRevInverseDataType=single
  Speed Measurement : mcbpositiondecoderlib/Speed Measurement  PositionUnit=Per unit  PositionScalingDatatype=uint32  SpeedCalculationMode=Time interval for speed calculation  SampleTimeAsync=Ts  MaximumApplicationSpeed=6000  SpeedResolution=5e-6  DelayLength=20  MaximumMeasurableSpeed=14999  MeasurableSpeedResolution=6.9849e-06  SpeedUnit=Per unit based on dialog  PerUnitSpeed=pmsm_motor2.N_base  SpeedDataType=dataType
  Theta_e : Outport  VectorParamsAs1DForOutWhenUnconnected=off
  speed : Outport  Port=2  VectorParamsAs1DForOutWhenUnconnected=off
  IndexFound : Outport  Port=3  InitialOutput=0  VectorParamsAs1DForOutWhenUnconnected=off
  wires:
  Mechanical to Electrical Position/1 -> Theta_e/1
  Speed Measurement/1 -> IIR Filter/1
  Quadrature Decoder/1 -> Speed Measurement/1, Mechanical to Electrical Position/1
  QEP_Position_Count/1 -> Quadrature Decoder/1
  Offset/1 -> Mechanical to Electrical Position/2
  IIR Filter/1 -> speed/1
  NOT/1 -> IndexFinder/Enable
  IndexFinder/1(Out1) -> Delay/1, IndexFound/1
  QEP_Index_Latch/1 -> IndexFinder/1(In1), Quadrature Decoder/2
  Delay/1 -> NOT/1

== system mcb_pmsm_foc_qep_dyno_f28069m_ADC/FOC Algorithm Motor2/Input Scaling/Calculate Phase Currents ==
  Ia_ADC : Inport
  Ib_ADC : Inport  Port=2
  Add : Sum  Inputs=-+
  Data Store Read : DataStoreRead  DataStoreName=IaOffset_motor2  IndexOptions=Index vector (dialog)  Indices=1  OutputSizes=1
  Data Store Read1 : DataStoreRead  DataStoreName=IbOffset_motor2  IndexOptions=Index vector (dialog)  Indices=1  OutputSizes=1
  Data Type Conversion : DataTypeConversion  OutDataTypeStr=int32  ConvertRealWorld=Stored Integer (SI)  SaturateOnIntegerOverflow=off  RndMeth=Floor
  Data Type Conversion1 : DataTypeConversion  OutDataTypeStr=dataType  SaturateOnIntegerOverflow=off  RndMeth=Floor
  Data Type Conversion3 : DataTypeConversion  OutDataTypeStr=fixdt(1,32,17)  ConvertRealWorld=Stored Integer (SI)  RndMeth=Simplest  SaturateOnIntegerOverflow=off
  Inverting / Non-inverting Current measurement amplifier : Gain  Gain=inverter_motor1.invertingAmp  RndMeth=Simplest  OutDataTypeStr=Inherit: Same as input
  Mux : Mux  Inputs=2
  Mux1 : Mux  Inputs=2
  Q17 per unit conversion : ArithShift  BitShiftNumber=-6
  Iab_meas_PU : Outport  VectorParamsAs1DForOutWhenUnconnected=off
  wires:
  Mux1/1 -> Add/1
  Data Type Conversion/1 -> Add/2
  Q17 per unit conversion/1 -> Data Type Conversion3/1
  Ia_ADC/1 -> Mux/1
  Add/1 -> Q17 per unit conversion/1
  Ib_ADC/1 -> Mux/2
  Mux/1 -> Data Type Conversion/1
  Data Type Conversion1/1 -> Inverting / Non-inverting Current measurement amplifier/1
  Data Type Conversion3/1 -> Data Type Conversion1/1
  Data Store Read/1 -> Mux1/1
  Data Store Read1/1 -> Mux1/2
  Inverting / Non-inverting Current measurement amplifier/1 -> Iab_meas_PU/1

== system mcb_pmsm_foc_qep_dyno_f28069m_ADC/Hardware Init/HW_Init/HW_Init (Codegen) ==
  note: System Outputs
  note: Block priorities are set to ensure the sequence of operation.
  note: for BoostXL-DRV8305 connected to LaunchXL-28069m
  Calibrate ADC offset for motor 1 current sensor : Subsystem  Priority=11  TreatAsAtomicUnit=on
  Calibrate ADC offset for motor 2 current sensor : Subsystem  Priority=12  TreatAsAtomicUnit=on
  Enable DRV8305 for motor 1 and motor 2 : Subsystem  Priority=10  TreatAsAtomicUnit=on

== system mcb_pmsm_foc_qep_dyno_f28069m_ADC/Hardware Init/HW_Init/HW_Init (sim) ==
  DRV830x Enable1 : Constant  OutDataTypeStr=boolean  SampleTime=-1
  Data Store Write : DataStoreWrite  DataStoreName=EnClosedLoop  IndexOptions=Index vector (dialog)  Indices=1  OutputSizes=1
  wires:
  DRV830x Enable1/1 -> Data Store Write/1

== system mcb_pmsm_foc_qep_dyno_f28069m_ADC/Motor1 and Motor2 coupled/Motor1_Measurements/Get_PU  ==
  rad : Inport
  Constant2 : Constant  Value=2*pi  OutDataTypeStr=single  SampleTime=-1
  Get_PU : Gain  Gain=1/(2*pi)  RndMeth=Simplest  OutDataTypeStr=Inherit: Same as input
  Mod : Math  Operator=mod
  PU : Outport  VectorParamsAs1DForOutWhenUnconnected=off
  wires:
  Get_PU/1 -> PU/1
  Mod/1 -> Get_PU/1
  Constant2/1 -> Mod/2
  rad/1 -> Mod/1

== system mcb_pmsm_foc_qep_dyno_f28069m_ADC/Motor1 and Motor2 coupled/Motor1_Measurements/Wrap ==
  in : Inport
  Constant2 : Constant  OutDataTypeStr=single  SampleTime=-1
  Mod : Math  Operator=mod
  out : Outport  VectorParamsAs1DForOutWhenUnconnected=off
  wires:
  Mod/1 -> out/1
  Constant2/1 -> Mod/2
  in/1 -> Mod/1

== system mcb_pmsm_foc_qep_dyno_f28069m_ADC/Motor1 and Motor2 coupled/Motor2_Measurements/Get_PU  ==
  rad : Inport
  Constant2 : Constant  Value=2*pi  OutDataTypeStr=single  SampleTime=-1
  Get_PU : Gain  Gain=1/(2*pi)  RndMeth=Simplest  OutDataTypeStr=Inherit: Same as input
  Mod : Math  Operator=mod
  PU : Outport  VectorParamsAs1DForOutWhenUnconnected=off
  wires:
  rad/1 -> Mod/1
  Constant2/1 -> Mod/2
  Mod/1 -> Get_PU/1
  Get_PU/1 -> PU/1

== system mcb_pmsm_foc_qep_dyno_f28069m_ADC/Motor1 and Motor2 coupled/Motor2_Measurements/Wrap ==
  in : Inport
  Constant2 : Constant  OutDataTypeStr=single  SampleTime=-1
  Mod : Math  Operator=mod
  out : Outport  VectorParamsAs1DForOutWhenUnconnected=off
  wires:
  in/1 -> Mod/1
  Constant2/1 -> Mod/2
  Mod/1 -> out/1

== system mcb_pmsm_foc_qep_dyno_f28069m_ADC/Serial Receive/Reference Signal/Data_Conditioning ==
  In1 : Inport
  Data Type Conversion1 : DataTypeConversion  OutDataTypeStr=single  RndMeth=Simplest  SaturateOnIntegerOverflow=off
  Data Type Conversion2 : DataTypeConversion  OutDataTypeStr=fixdt(1,16,12)  ConvertRealWorld=Stored Integer (SI)  RndMeth=Simplest  SaturateOnIntegerOverflow=off
  Demux : Demux  Outputs=2
  Logical signal : Outport  VectorParamsAs1DForOutWhenUnconnected=off
  PU_data : Outport  Port=2  VectorParamsAs1DForOutWhenUnconnected=off
  wires:
  Data Type Conversion1/1 -> PU_data/1
  Data Type Conversion2/1 -> Data Type Conversion1/1
  In1/1 -> Demux/1
  Demux/1 -> Data Type Conversion2/1
  Demux/2 -> Logical signal/1

== system mcb_pmsm_foc_qep_dyno_f28069m_ADC/Serial Receive/Reference Signal/If Action Subsystem ==
  In1 : Inport
  Action Port : ActionPort  ActionPortLabel=if(u1 == 1)
  Data Store Write2 : DataStoreWrite  DataStoreName=SpeedRef  IndexOptions=Index vector (dialog)  Indices=1  OutputSizes=1
  Data Type Conversion1 : DataTypeConversion  OutDataTypeStr=dataType  RndMeth=Simplest  SaturateOnIntegerOverflow=off
  wires:
  Data Type Conversion1/1 -> Data Store Write2/1
  In1/1 -> Data Type Conversion1/1

== system mcb_pmsm_foc_qep_dyno_f28069m_ADC/Serial Receive/Reference Signal/If Action Subsystem1 ==
  In1 : Inport
  Action Port : ActionPort  ActionPortLabel=elseif(u1 == 2)
  Data Store Write2 : DataStoreWrite  DataStoreName=IqRef  IndexOptions=Index vector (dialog)  Indices=1  OutputSizes=1
  Data Type Conversion2 : DataTypeConversion  OutDataTypeStr=dataType  RndMeth=Simplest  SaturateOnIntegerOverflow=off
  wires:
  In1/1 -> Data Type Conversion2/1
  Data Type Conversion2/1 -> Data Store Write2/1

== system mcb_pmsm_foc_qep_dyno_f28069m_ADC/Serial Receive/Reference Signal/If Action Subsystem2 ==
  In1 : Inport
  Action Port : ActionPort  ActionPortLabel=elseif( u1 == 0)
  Data Store Write2 : DataStoreWrite  DataStoreName=SpeedRef  IndexOptions=Index vector (dialog)  Indices=1  OutputSizes=1
  Data Type Conversion1 : DataTypeConversion  OutDataTypeStr=dataType  RndMeth=Simplest  SaturateOnIntegerOverflow=off
  wires:
  Data Type Conversion1/1 -> Data Store Write2/1
  In1/1 -> Data Type Conversion1/1

== system mcb_pmsm_foc_qep_dyno_f28069m_ADC/Serial Receive/Reference Signal/unParse ==
  Data : Inport
  Bitwise Operator : simulink/Logic and Bit Operations/Bitwise Operator  logicop=AND  UseBitMask=on  BitMask=hex2dec('0001')  BitMaskRealWorld=Stored Integer
  Bitwise Operator1 : simulink/Logic and Bit Operations/Bitwise Operator  logicop=AND  UseBitMask=on  BitMask=hex2dec('00F0')  BitMaskRealWorld=Stored Integer
  Bitwise Operator2 : simulink/Logic and Bit Operations/Bitwise Operator  logicop=AND  UseBitMask=on  BitMask=hex2dec('0006')  BitMaskRealWorld=Stored Integer
  Data Type Conversion3 : DataTypeConversion  OutDataTypeStr=boolean  RndMeth=Simplest  SaturateOnIntegerOverflow=off
  Data Type Conversion4 : DataTypeConversion  OutDataTypeStr=uint16  RndMeth=Simplest  SaturateOnIntegerOverflow=off
  Data Type Conversion5 : DataTypeConversion  OutDataTypeStr=uint16  RndMeth=Simplest  SaturateOnIntegerOverflow=off
  Shift Arithmetic : ArithShift  BitShiftNumber=1
  Shift Arithmetic1 : ArithShift  BitShiftNumber=4
  Enable_PWM : Outport
  Motor1/2 : Outport  Port=2
  Debug_sig : Outport  Port=3
  wires:
  Bitwise Operator2/1 -> Shift Arithmetic/1
  Bitwise Operator1/1 -> Shift Arithmetic1/1
  Data/1 -> Bitwise Operator/1, Bitwise Operator2/1, Bitwise Operator1/1
  Bitwise Operator/1 -> Data Type Conversion3/1
  Shift Arithmetic1/1 -> Data Type Conversion4/1
  Data Type Conversion3/1 -> Enable_PWM/1
  Shift Arithmetic/1 -> Data Type Conversion5/1
  Data Type Conversion5/1 -> Motor1/2/1
  Data Type Conversion4/1 -> Debug_sig/1

== system mcb_pmsm_foc_qep_dyno_f28069m_ADC/Serial Receive/Simulation/Data_Conditioning ==
  In1 : Inport
  Data Type Conversion1 : DataTypeConversion  OutDataTypeStr=single  RndMeth=Simplest  SaturateOnIntegerOverflow=off
  Data Type Conversion2 : DataTypeConversion  OutDataTypeStr=fixdt(1,16,12)  ConvertRealWorld=Stored Integer (SI)  RndMeth=Simplest  SaturateOnIntegerOverflow=off
  Out1 : Outport  VectorParamsAs1DForOutWhenUnconnected=off
  wires:
  Data Type Conversion1/1 -> Out1/1
  Data Type Conversion2/1 -> Data Type Conversion1/1
  In1/1 -> Data Type Conversion2/1

== system mcb_pmsm_foc_qep_dyno_f28069m_ADC/FOC Algorithm Motor1/Control_System/Open Loop Start-Up/Ramp Generator ==
  Ramp_Time : Inport
  Enable : Inport  Port=2
  Divide : Product  Inputs=*/  RndMeth=Simplest  OutDataTypeStr=Inherit: Same as first input
  NOT : Logic  Operator=NOT  IconShape=distinctive  AllPortsSameDT=off  OutDataTypeStr=boolean
  One : Constant  OutDataTypeStr=dataType  SampleTime=-1
  Ramp Generator : DiscreteIntegrator  IntegratorMethod=Accumulation: Forward Euler  gainval=1  ExternalReset=sampled level  SampleTime=-1  OutDataTypeStr=dataType  RndMeth=Simplest  LimitOutput=on  UpperSaturationLimit=1  LowerSaturationLimit=0  ICPrevOutput=DiscIntNeverNeededParam  ICPrevScaledInput=DiscIntNeverNeededParam
  Sample_Time : Gain  Gain=Ts  RndMeth=Simplest  OutDataTypeStr=Inherit: Same as input
  Ramp : Outport
  wires:
  Divide/1 -> Sample_Time/1
  Ramp Generator/1 -> Ramp/1  "Eps"
  Sample_Time/1 -> Ramp Generator/1
  One/1 -> Divide/1
  Ramp_Time/1 -> Divide/2
  Enable/1 -> NOT/1
  NOT/1 -> Ramp Generator/2

== system mcb_pmsm_foc_qep_dyno_f28069m_ADC/FOC Algorithm Motor1/Input Scaling/ Calculate Speed/IndexFinder ==
  In1 : Inport
  Enable : EnablePort
  AND : Logic  AllPortsSameDT=off  OutDataTypeStr=boolean
  Compare To Constant : simulink/Logic and Bit Operations/Compare To Constant  relop===  const=0  OutDataTypeStr=boolean
  Compare To Constant1 : simulink/Logic and Bit Operations/Compare To Constant  relop=>  const=0  OutDataTypeStr=boolean
  Delay3 : Delay  DelayLength=1
  Out1 : Outport
  wires:
  In1/1 -> Delay3/1, Compare To Constant1/1
  Compare To Constant1/1 -> AND/2
  Compare To Constant/1 -> AND/1
  Delay3/1 -> Compare To Constant/1
  AND/1 -> Out1/1

== system mcb_pmsm_foc_qep_dyno_f28069m_ADC/FOC Algorithm Motor1/SCI (Code Generation)/Data_Logging/Data ==
  Data : Inport
  Data_width : Inport  Port=2
  Action Port : ActionPort  ActionPortLabel=else
  Mux : Mux  Inputs=2
  Start : Constant  Value=hex2dec('0000')  OutDataTypeStr=uint16
  Data_out : Outport  VectorParamsAs1DForOutWhenUnconnected=off
  Iteration : Outport  Port=2  VectorParamsAs1DForOutWhenUnconnected=off
  wires:
  Start/1 -> Mux/2
  Mux/1 -> Data_out/1
  Data/1 -> Mux/1
  Data_width/1 -> Iteration/1

== system mcb_pmsm_foc_qep_dyno_f28069m_ADC/FOC Algorithm Motor1/SCI (Code Generation)/Data_Logging/Data_Conditioning ==
  In1 : Inport
  Data Type Conversion : DataTypeConversion  OutDataTypeStr=fixdt(1,16,12)  RndMeth=Simplest  SaturateOnIntegerOverflow=off
  Data Type Conversion3 : DataTypeConversion  OutDataTypeStr=uint16  ConvertRealWorld=Stored Integer (SI)  SaturateOnIntegerOverflow=off  RndMeth=Floor
  Out1 : Outport  VectorParamsAs1DForOutWhenUnconnected=off
  wires:
  In1/1 -> Data Type Conversion/1
  Data Type Conversion3/1 -> Out1/1
  Data Type Conversion/1 -> Data Type Conversion3/1

== system mcb_pmsm_foc_qep_dyno_f28069m_ADC/FOC Algorithm Motor1/SCI (Code Generation)/Data_Logging/End ==
  Data : Inport
  Data_width : Inport  Port=2
  Action Port : ActionPort  ActionPortLabel=elseif(u1 == 599)
  Bias : Bias  Bias=1  SaturateOnIntegerOverflow=off
  Mux : Mux  Inputs=2
  Start : Constant  Value=hex2dec('4545')  OutDataTypeStr=uint16
  Data_out : Outport  VectorParamsAs1DForOutWhenUnconnected=off
  Iteration : Outport  Port=2  VectorParamsAs1DForOutWhenUnconnected=off
  wires:
  Mux/1 -> Data_out/1
  Data_width/1 -> Bias/1
  Start/1 -> Mux/2
  Bias/1 -> Iteration/1
  Data/1 -> Mux/1

== system mcb_pmsm_foc_qep_dyno_f28069m_ADC/FOC Algorithm Motor1/SCI (Code Generation)/Data_Logging/Start ==
  Data : Inport
  Data_width : Inport  Port=2
  Action Port : ActionPort  ActionPortLabel=if(u1 == 0)
  Bias : Bias  Bias=1  SaturateOnIntegerOverflow=off
  End : Constant  Value=hex2dec('5353')  OutDataTypeStr=uint16
  Mux : Mux  Inputs=2
  Data_out : Outport  VectorParamsAs1DForOutWhenUnconnected=off
  Iteration : Outport  Port=2  VectorParamsAs1DForOutWhenUnconnected=off
  wires:
  End/1 -> Mux/1
  Mux/1 -> Data_out/1
  Data_width/1 -> Bias/1
  Bias/1 -> Iteration/1
  Data/1 -> Mux/2

== system mcb_pmsm_foc_qep_dyno_f28069m_ADC/FOC Algorithm Motor2/Enable Motor2 after a delay/Delay to start motor1 (codegen)/Disable EnMtr2TrqCtrl ==
  Enable : EnablePort  StatesWhenEnabling=reset
  Constant : Constant  Value=0  OutDataTypeStr=boolean
  Data Store Write : DataStoreWrite  DataStoreName=EnMtr2TrqCtrl  IndexOptions=Index vector (dialog)  Indices=1  OutputSizes=1
  wires:
  Constant/1 -> Data Store Write/1

== system mcb_pmsm_foc_qep_dyno_f28069m_ADC/FOC Algorithm Motor2/Enable Motor2 after a delay/Delay to start motor1 (codegen)/Enable EnMtr2TrqCtrl after 2 sec delay ==
  Enable : EnablePort  StatesWhenEnabling=reset
  Add : Sum
  Constant : Constant  OutDataTypeStr=boolean
  Constant1 : Constant  Value=0  OutDataTypeStr=boolean
  Constant2 : Constant  OutDataTypeStr=uint32
  Enable EnMtr2TrqCtrl : Subsystem  TreatAsAtomicUnit=on
  Switch : Switch  Criteria=u2 > Threshold  Threshold=40000  SaturateOnIntegerOverflow=off  InputSameDT=off
  Unit Delay : UnitDelay  SampleTime=-1  HasFrameUpgradeWarning=on
  wires:
  Constant1/1 -> Switch/3
  Constant/1 -> Switch/1
  Constant2/1 -> Add/1
  Add/1 -> Unit Delay/1, Switch/2
  Unit Delay/1 -> Add/2
  Switch/1 -> Enable EnMtr2TrqCtrl/Enable

== system mcb_pmsm_foc_qep_dyno_f28069m_ADC/FOC Algorithm Motor2/Enable Motor2 after a delay/Delay to start motor2 (sim)/Delay 0.5 sec ==
  Enable : EnablePort  StatesWhenEnabling=reset
  Add : Sum
  Constant : Constant  OutDataTypeStr=boolean
  Constant1 : Constant  Value=0  OutDataTypeStr=boolean
  Constant2 : Constant  OutDataTypeStr=uint32
  Switch : Switch  Criteria=u2 > Threshold  Threshold=10000  SaturateOnIntegerOverflow=off  InputSameDT=off
  Unit Delay : UnitDelay  SampleTime=-1  HasFrameUpgradeWarning=on
  Out1 : Outport
  wires:
  Constant1/1 -> Switch/3
  Constant/1 -> Switch/1
  Constant2/1 -> Add/1
  Add/1 -> Unit Delay/1, Switch/2
  Unit Delay/1 -> Add/2
  Switch/1 -> Out1/1

== system mcb_pmsm_foc_qep_dyno_f28069m_ADC/FOC Algorithm Motor2/Enable Motor2 after a delay/Delay to start motor2 (sim)/Enabled Subsystem ==
  Enable : EnablePort
  Constant : Constant  OutDataTypeStr=boolean
  Data Store Write : DataStoreWrite  DataStoreName=EnMtr2TrqCtrl  IndexOptions=Index vector (dialog)  Indices=1  OutputSizes=1
  wires:
  Constant/1 -> Data Store Write/1

== system mcb_pmsm_foc_qep_dyno_f28069m_ADC/FOC Algorithm Motor2/Enable Motor2 after a delay/Delay to start motor2 (sim)/Enabled Subsystem2 ==
  Enable : EnablePort
  Constant : Constant  Value=0  OutDataTypeStr=boolean
  Data Store Write : DataStoreWrite  DataStoreName=EnMtr2TrqCtrl  IndexOptions=Index vector (dialog)  Indices=1  OutputSizes=1
  wires:
  Constant/1 -> Data Store Write/1

== system mcb_pmsm_foc_qep_dyno_f28069m_ADC/FOC Algorithm Motor2/Input Scaling/ Calculate Speed/IndexFinder ==
  In1 : Inport
  Enable : EnablePort
  AND : Logic  AllPortsSameDT=off  OutDataTypeStr=boolean
  Compare To Constant : simulink/Logic and Bit Operations/Compare To Constant  relop===  const=0  OutDataTypeStr=boolean
  Compare To Constant1 : simulink/Logic and Bit Operations/Compare To Constant  relop=>  const=0  OutDataTypeStr=boolean
  Delay3 : Delay  DelayLength=1
  Out1 : Outport
  wires:
  In1/1 -> Delay3/1, Compare To Constant1/1
  Compare To Constant1/1 -> AND/2
  Compare To Constant/1 -> AND/1
  Delay3/1 -> Compare To Constant/1
  AND/1 -> Out1/1

== system mcb_pmsm_foc_qep_dyno_f28069m_ADC/Hardware Init/HW_Init/HW_Init (Codegen)/Calibrate ADC offset for motor 1 current sensor ==
  note: Enable ADC offset calibration only when motor is not loaded and not rotating due to external factors
  ADC Calib Enable : Constant  Value=inverter_motor1.ADCOffsetCalibEnable  OutDataTypeStr=Inherit: Inherit via back propagation
  Calculate ADC Offset : Subsystem  Priority=1001  TreatAsAtomicUnit=on
  Default ADC Offset : Subsystem  Priority=1001  TreatAsAtomicUnit=on
  NOT : Logic  Operator=NOT  IconShape=distinctive  AllPortsSameDT=off  OutDataTypeStr=boolean
  wires:
  NOT/1 -> Default ADC Offset/Enable
  ADC Calib Enable/1 -> Calculate ADC Offset/Enable, NOT/1

== system mcb_pmsm_foc_qep_dyno_f28069m_ADC/Hardware Init/HW_Init/HW_Init (Codegen)/Calibrate ADC offset for motor 2 current sensor ==
  note: Enable ADC offset calibration only when motor is not loaded and not rotating due to external factors
  ADC Calib Enable : Constant  Value=inverter_motor2.ADCOffsetCalibEnable  OutDataTypeStr=Inherit: Inherit via back propagation
  Calculate ADC Offset : Subsystem  Priority=1001  TreatAsAtomicUnit=on
  Default ADC Offset : Subsystem  Priority=1001  TreatAsAtomicUnit=on
  NOT : Logic  Operator=NOT  IconShape=distinctive  AllPortsSameDT=off  OutDataTypeStr=boolean
  wires:
  ADC Calib Enable/1 -> Calculate ADC Offset/Enable, NOT/1
  NOT/1 -> Default ADC Offset/Enable
